simulink model "test_monoaxial"  (R2023a)
settings: Solver=FixedStepAuto  StartTime=0.0  StopTime=inf  FixedStep=0.01  RelTol=1e-3  EnableMultiTasking=on
values from neighbouring files (symbols this model uses):
  A = [Ts 0;Ts Ts]    [monoaxial.m]
  B = [1;0]    [monoaxial.m]
  C = [1,0]    [monoaxial.m]
  D = 0    [monoaxial.m]
undefined symbols (not defined in the file or in its folder): dev, Discrete, Main, pwm_output0, Time
libraries: px4Sensorslib x4, px4lib x1, px4uORBlib x1, ctrlSharedLib x1, slpidlib x1
settings Model: SimulationMode=external  ExtModeTrigDuration=10  Creator=ArriGE66  LastModifiedBy=User
settings SolverCC: PositivePriorityOrder=on
settings OptimizationCC: EnhancedBackFolding=on  PassReuseOutputArgsAs=Individual arguments  ZeroExternalMemoryAtStartup=off  ZeroInternalMemoryAtStartup=off  MaxStackSize=64  OptimizeBlockOrder=speed  DifferentSizesBufferReuse=on  OptimizationCustomize=off  EfficientTunableParamExpr=on
settings DebuggingCC: ParameterTunabilityLossMsg=error
settings HardwareCC: ProdBitPerPointer=32  ProdBitPerSizeT=32  ProdBitPerPtrDiffT=32  ProdLargestAtomicInteger=Long  ProdLargestAtomicFloat=Double  ProdWordSize=32  ProdLongLongMode=on  ProdHWDeviceType=ARM Compatible->ARM Cortex
settings SFSimCC: MATLABDynamicMemAlloc=off  SimTargetLang=C++
settings RTWCC: Description=Embedded Coder  SystemTargetFile=ert.tlc  HardwareBoard=PX4 Cube Orange  TemplateMakefile=ert_default_tmf  Toolchain=GNU Tools for PX4 Autopilots  TargetLang=C++
settings CodeAppCC: ForceParamTrailComments=on  IgnoreCustomStorageClasses=off  OperatorAnnotations=on  SimulinkDataObjDesc=on  SFDataObjDesc=on  InsertBlockDesc=on
settings ERTTargetCC: ExtMode=on  ExtModeTransport=3  ExtModeStaticAlloc=on  ExtModeStaticAllocSize=1024  ExtModeMexFile=ext_xcp  ExtModeMexArgs=1 COM10 3000000  ExtModeIntrfLevel=Level2 - Open

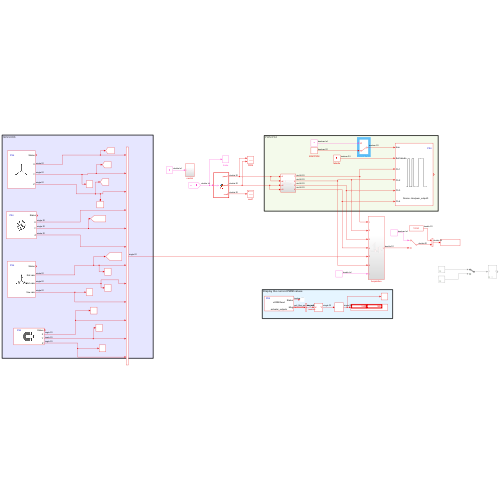
[thumbnail: Simulink's stored preview of the top-level diagram]
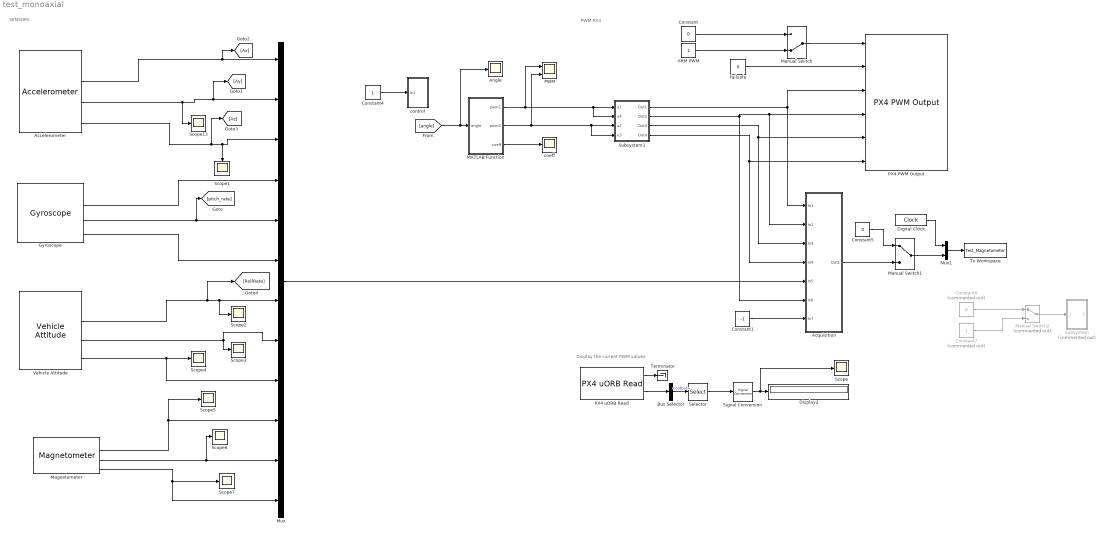
== system test_monoaxial ==
  note: PWM PX4
  note: SENSORS
  note: Display the current PWM values
  ARM PWM : Constant  OutDataTypeStr=boolean  SampleTime=0.01
  Accelerometer : px4Sensorslib/Accelerometer  uorbTimeStamp=off  BlockingMode=off  BlockTimeout=1e-3  sampleTime=1/100
  Acquisition : Subsystem
  Angle : Scope
  Bus Selector : BusSelector  OutputSignals=output
  Constant : Constant  Value=0  OutDataTypeStr=boolean
  Constant1 : Constant  Value=-1
  Constant4 : Constant
  Constant5 : Constant  Value=0  OutDataTypeStr=boolean
  Constant6 : Constant  Commented=on  Value=0
  Constant7 : Constant  Commented=on
  Digital Clock : DigitalClock  SampleTime=-1
  Display2 : Display
  Gyroscope : px4Sensorslib/Gyroscope  uorbTimeStamp=off  BlockingMode=off  BlockTimeout=1e-3  sampleTime=1/100
  MATLAB Function : MATLAB Function  TreatAsAtomicUnit=on
  Magnetometer : px4Sensorslib/Magnetometer  uorbTimeStamp=off  BlockingMode=off  BlockTimeout=1e-3  sampleTime=0.01
  Manual Switch : ManualSwitch  CurrentSetting=0
  Manual Switch1 : ManualSwitch
  Manual Switch2 : ManualSwitch  Commented=on
  Mux : Mux  Inputs=12
  Mux1 : Mux  Inputs=2
  PWM : Scope  NumInputPorts=2
  PX4 PWM Output : px4lib/PX4 PWM Output  pwmDevice=Main (/dev/pwm_output0)  pwmChannel1_=on  pwmChannel2_=on  pwmChannel3_=on  pwmChannel4_=on  pwmChannel5_=off  pwmChannel6_=off  pwmChannel7_=off  pwmChannel8_=off  forceTerminateFailsafe=off  outputErrorStatus=on
  PX4 uORB Read : px4uORBlib/PX4 uORB Read  uORBTopic=actuator_outputs  selectInstance=actuator_outputs  SampleTime=0.01  BlockingMode=off  BlockTimeout=1e-3
  Scope{,1..7,13} (9 alike) : Scope
  Selector : Selector  InputPortWidth=16  IndexOptions=Index vector (dialog)  Indices=[1 2]  OutputSizes=1
  Signal Conversion : SignalConversion  OverrideOpt=off
  Subsystem : Subsystem  Commented=on  mask{delta_t=10}
      mask prompts: delta_t "delta_time [s]"
  Subsystem1 : Subsystem
  Terminator : Terminator
  To Workspace : ToWorkspace  VariableName=Test_Magnetometer  SampleTime=-1
      settings: Save2DSignal=2-D array (concatenate along first dimension)
  Vehicle Attitude : px4Sensorslib/Vehicle Attitude  rollRate=on  pitchRate=on  yawRate=on  quaternion=off  uorbTimeStamp=off  BlockingMode=off  BlockTimeout=0.001  sampleTime=1/100
  coeff : Scope
  control : Subsystem
  failsafe : Constant  Value=0  OutDataTypeStr=boolean  SampleTime=0.01
  wires:
  Manual Switch/1 -> PX4 PWM Output/1
  Bus Selector/1 -> Selector/1  "<output>"
  PX4 uORB Read/1 -> Terminator/1
  failsafe/1 -> PX4 PWM Output/2
  Selector/1 -> Signal Conversion/1
  PX4 uORB Read/2 -> Bus Selector/1
  Signal Conversion/1 -> Scope/1, Display2/1
  Vehicle Attitude/3 -> Scope3/1, Mux/8
  Vehicle Attitude/2 -> [RollRate], Scope2/1, Mux/7
  ARM PWM/1 -> Manual Switch/2
  Constant/1 -> Manual Switch/1
  Gyroscope/4 -> Mux/6
  Gyroscope/3 -> [pitch_rate], Mux/5
  Gyroscope/2 -> Mux/4
  Accelerometer/2 -> [Ax], Mux/1
  Accelerometer/3 -> Scope13/1, [Ay], Mux/2
  Accelerometer/4 -> [Az], Mux/3, Scope1/1
  Mux/1 -> Acquisition/5(In5)
  Acquisition/1(Out1) -> Manual Switch1/2
  Constant5/1 -> Manual Switch1/1
  Mux1/1 -> To Workspace/1
  Digital Clock/1 -> Mux1/1
  Manual Switch1/1 -> Mux1/2
  Constant7/1 -> Manual Switch2/2
  Constant6/1 -> Manual Switch2/1
  Manual Switch2/1 -> Subsystem/1(In1)
  Vehicle Attitude/4 -> Mux/9, Scope4/1
  Subsystem1/2(Out2) -> Acquisition/6(In6), Acquisition/2(In2), PX4 PWM Output/4
  Subsystem1/3(Out3) -> Acquisition/3(In3), PX4 PWM Output/5
  Subsystem1/1(Out1) -> Acquisition/1(In1), PX4 PWM Output/3
  Subsystem1/4(Out4) -> Acquisition/4(In4), PX4 PWM Output/6
  Magnetometer/2 -> Mux/10, Scope5/1
  Magnetometer/3 -> Mux/11, Scope6/1
  Magnetometer/4 -> Mux/12, Scope7/1
  Constant1/1 -> Acquisition/7(In7)
  [angle] -> MATLAB Function/1(angle), Angle/1
  MATLAB Function/1(pwm1) -> Subsystem1/2(u4), Subsystem1/1(u1), PWM/1
  MATLAB Function/3(coeff) -> coeff/1
  Constant4/1 -> control/1(In1)
  MATLAB Function/2(pwm2) -> Subsystem1/4(u3), Subsystem1/3(u2), PWM/2

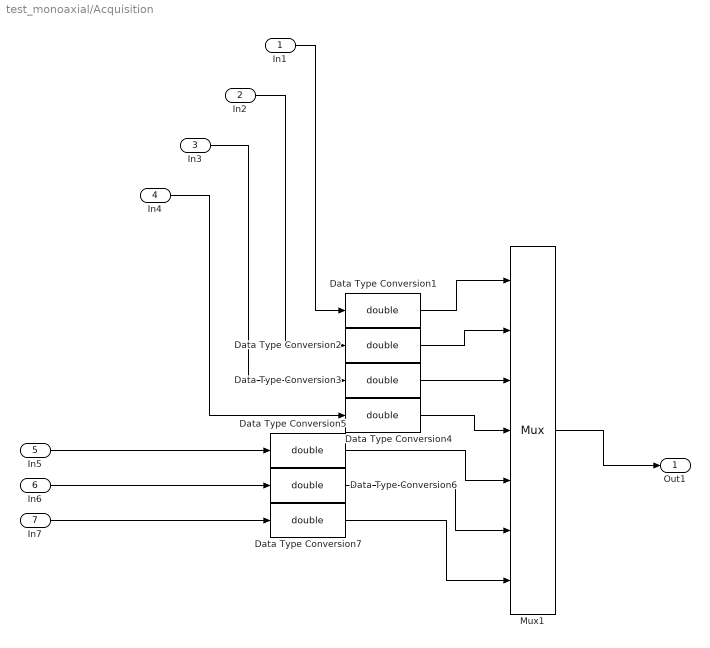
== system test_monoaxial/Acquisition ==
  In1 : Inport
  In2 : Inport  Port=2
  In3 : Inport  Port=3
  In4 : Inport  Port=4
  In5 : Inport  Port=5
  In6 : Inport  Port=6
  In7 : Inport  Port=7
  Data Type Conversion{1..7} (7 alike) : DataTypeConversion  OutDataTypeStr=double  SaturateOnIntegerOverflow=off  RndMeth=Floor
  Mux1 : Mux  Inputs=7
      settings: DisplayOption=signals
  Out1 : Outport
  wires:
  In7/1 -> Data Type Conversion7/1
  In2/1 -> Data Type Conversion2/1
  Data Type Conversion1/1 -> Mux1/1
  Data Type Conversion7/1 -> Mux1/7
  Data Type Conversion3/1 -> Mux1/3
  Data Type Conversion5/1 -> Mux1/5
  Data Type Conversion4/1 -> Mux1/4
  Data Type Conversion2/1 -> Mux1/2
  Data Type Conversion6/1 -> Mux1/6
  In3/1 -> Data Type Conversion3/1
  In6/1 -> Data Type Conversion6/1
  Mux1/1 -> Out1/1
  In5/1 -> Data Type Conversion5/1
  In1/1 -> Data Type Conversion1/1
  In4/1 -> Data Type Conversion4/1

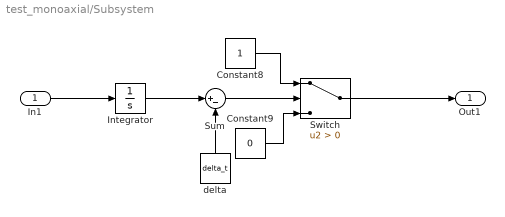
== system test_monoaxial/Subsystem ==
  In1 : Inport
  Constant8 : Constant
  Constant9 : Constant  Value=0
  Integrator : Integrator
  Sum : Sum  Inputs=|+-
  Switch : Switch  Criteria=u2 > Threshold  SaturateOnIntegerOverflow=off  InputSameDT=off
  delta : Constant  Value=delta_t
  Out1 : Outport
  wires:
  delta/1 -> Sum/2
  In1/1 -> Integrator/1
  Sum/1 -> Switch/2
  Integrator/1 -> Sum/1
  Switch/1 -> Out1/1
  Constant9/1 -> Switch/3
  Constant8/1 -> Switch/1

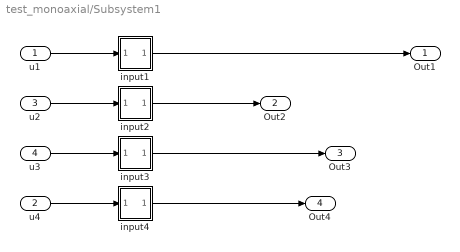
== system test_monoaxial/Subsystem1 ==
  u1 : Inport
  u4 : Inport  Port=2
  u2 : Inport  Port=3
  u3 : Inport  Port=4
  input1 : Subsystem
  input2 : Subsystem
  input3 : Subsystem
  input4 : Subsystem
  Out1 : Outport
  Out2 : Outport  Port=2
  Out3 : Outport  Port=3
  Out4 : Outport  Port=4
  wires:
  u2/1 -> input2/1(In1)
  u1/1 -> input1/1(In1)
  input1/1(Out1) -> Out1/1
  u4/1 -> input4/1(In1)
  input4/1(Out1) -> Out4/1
  input2/1(Out1) -> Out2/1
  u3/1 -> input3/1(In1)
  input3/1(Out1) -> Out3/1

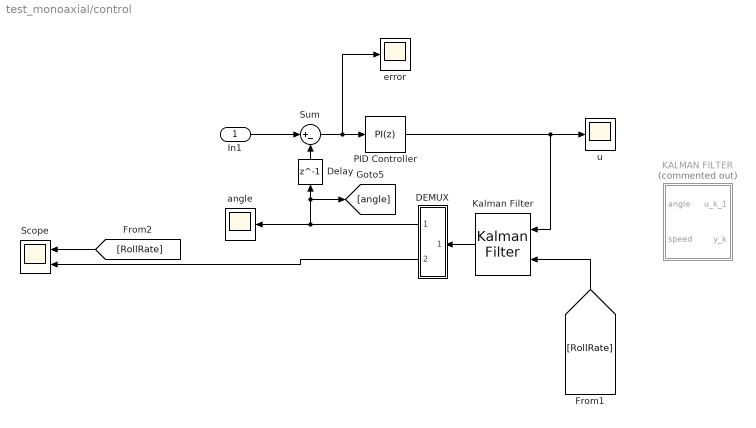
== system test_monoaxial/control ==
  In1 : Inport
  DEMUX : MATLAB Function  TreatAsAtomicUnit=on
  Delay : Delay  DelayLength=1
  KALMAN FILTER : Subsystem  Commented=on
  Kalman Filter : ctrlSharedLib/Kalman Filter  TimeDomain=Discrete-Time  UseCurrentEstimator=on  ModelSource=Individual A, B, C, D matrices  ModelSourceVariable=ss(0.95,1,1,0,1)  A=A  B=B  C=C  D=D  NumberOfStates=1  NumberOfInputs=1  NumberOfOutputs=1  InitialEstimateSource=Dialog  X0=0  P0=10  UseK=off  UseGH=off  NumberOfProcessNoiseInputs=1  G=1  TimeInvariantG=on  H=0  TimeInvariantH=on  Q=10  TimeInvariantQ=on  R=0.01  TimeInvariantR=on  N=0  TimeInvariantN=on  AddInputPort=on  AddEnablePort=off  OutputEstimatedY=off  OutputP=off  Ts=-1
  PID Controller : slpidlib/PID Controller  Controller=PI  Form=Parallel  TimeDomain=Discrete-time  UseExternalTs=off  SampleTime=-1  IntegratorMethod=Forward Euler  FilterMethod=Forward Euler  ControllerParametersSource=internal  P=14.044  I=209.05  UseKiTs=off  D=0  N=100  UseFilter=on  TunerSelectOption=Transfer Function Based (PID Tuner App)  InitialConditionSource=internal  InitialConditionForIntegrator=0  InitialConditionForFilter=0  DifferentiatorICPrevScaledInput=0  ExternalReset=none  TrackingMode=off  Kt=1  LimitOutput=off  SatLimitsSource=internal  UpperSaturationLimit=inf  LowerSaturationLimit=-inf  LinearizeAsGain=on  AntiWindupMode=none  Kb=1  LimitIntegrator=off  UpperIntegratorSaturationLimit=inf  LowerIntegratorSaturationLimit=-inf  POutMin=[]  POutMax=[]  IOutMin=[]  IOutMax=[]  DOutMin=[]  DOutMax=[]  NOutMin=[]  NOutMax=[]  SumOutMin=[]  SumOutMax=[]  SaturationOutMin=[]  SaturationOutMax=[]  PParamMin=[]  PParamMax=[]  IParamMin=[]  IParamMax=[]  DParamMin=[]  DParamMax=[]  NParamMin=[]  NParamMax=[]  KbParamMin=[]  KbParamMax=[]  KtParamMin=[]  KtParamMax=[]  KbOutMin=[]  KbOutMax=[]  KtOutMin=[]  KtOutMax=[]  IntegratorOutMin=[]  IntegratorOutMax=[]  FilterOutMin=[]  FilterOutMax=[]  SumI1OutMin=[]  SumI1OutMax=[]  SumI2OutMin=[]  SumI2OutMax=[]  SumI3OutMin=[]  SumI3OutMax=[]  SumI4OutMin=[]  SumI4OutMax=[]  SumDOutMin=[]  SumDOutMax=[]  DifferentiatorOutMin=[]  DifferentiatorOutMax=[]  FilterDiffOutCoefMin=[]  FilterDiffOutCoefMax=[]  ReciprocalOutMin=[]  ReciprocalOutMax=[]  SumDenOutMin=[]  SumDenOutMax=[]  SumNumOutMin=[]  SumNumOutMax=[]  DivideOutMin=[]  DivideOutMax=[]  UdiffTsProdOutMin=[]  UdiffTsProdOutMax=[]  NTsProdOutMin=[]  NTsProdOutMax=[]  UintegralTsProdOutMin=[]  UintegralTsProdOutMax=[]  UngainTsProdOutMin=[]  UngainTsProdOutMax=[]  ClampingZeroOutDataTypeStr=Inherit: Inherit via back propagation  ClampingZeroOutMin=[]  ClampingZeroOutMax=[]  FilterDenConstantOutDataTypeStr=Inherit: Inherit via back propagation  FilterDenConstantOutMin=[]  FilterDenConstantOutMax=[]  PCopyOutDataTypeStr=Inherit: Inherit via back propagation  PCopyOutMin=[]  PCopyOutMax=[]  NCopyOutDataTypeStr=Inherit: Inherit via back propagation  NCopyOutMin=[]  NCopyOutMax=[]  IntegratorContinuousStateAttributes=''  IntegratorStateMustResolveToSignalObject=off  IntegratorRTWStateStorageClass=Auto  FilterContinuousStateAttributes=''  FilterStateMustResolveToSignalObject=off  FilterRTWStateStorageClass=Auto  ParallelPVariant=InternalParameters  IdealPVariant=Disabled  IVariant=InternalParameters  DVariant=Disabled  IntegratorVariant=Discrete  SatVariant=Disabled  AWVariant=Passthrough  PCopyVariant=Disabled  TRVariant=Disabled  FdbkBlocksVariant=Forward  IdealPFdbkVariant=Disabled  SatFdbkVariant=Disabled  DerivativeFilterVariant=Disabled  NVariant=Disabled  NCopyVariant=Disabled_SignalSpec  FilterICVariant=Disabled  IntegratorICVariant=InternalICs  ExternalResetVariant=Disabled  TRSumVariant=Passthrough  SumFdbkVariant=Disabled  SumVariant=Sum_PI  TsampFilterVariant=InternalTs  TsampNgainVariant=Passthrough  TsampIntegralVariant=Disabled_SignalSpec  ExternalSaturationOutDataTypeStr=Inherit: Same as second input
  Scope : Scope  NumInputPorts=2
  Sum : Sum  Inputs=|+-
  angle : Scope
  error : Scope
  u : Scope
  wires:
  Sum/1 -> error/1, PID Controller/1
  DEMUX/1(angle) -> angle/1, Delay/1, [angle]
  In1/1 -> Sum/1
  PID Controller/1 -> Kalman Filter/1, u/1
  [RollRate] -> Scope/1
  DEMUX/2(speed) -> Scope/2
  [RollRate] -> Kalman Filter/2
  Delay/1 -> Sum/2
  Kalman Filter/1 -> DEMUX/1(x)

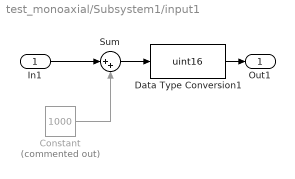
== system test_monoaxial/Subsystem1/input1 ==
  In1 : Inport
  Constant : Constant  Commented=on  Value=1000  SampleTime=0.01
  Data Type Conversion1 : DataTypeConversion  OutDataTypeStr=uint16  SaturateOnIntegerOverflow=off  RndMeth=Floor
  Sum : Sum  Inputs=|++
  Out1 : Outport
  wires:
  Sum/1 -> Data Type Conversion1/1
  In1/1 -> Sum/1
  Constant/1 -> Sum/2
  Data Type Conversion1/1 -> Out1/1

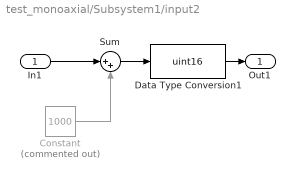
== system test_monoaxial/Subsystem1/input2 ==
  In1 : Inport
  Constant : Constant  Commented=on  Value=1000  SampleTime=0.01
  Data Type Conversion1 : DataTypeConversion  OutDataTypeStr=uint16  SaturateOnIntegerOverflow=off  RndMeth=Floor
  Sum : Sum  Inputs=|++
  Out1 : Outport
  wires:
  Sum/1 -> Data Type Conversion1/1
  In1/1 -> Sum/1
  Constant/1 -> Sum/2
  Data Type Conversion1/1 -> Out1/1

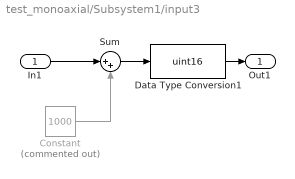
== system test_monoaxial/Subsystem1/input3 ==
  In1 : Inport
  Constant : Constant  Commented=on  Value=1000  SampleTime=0.01
  Data Type Conversion1 : DataTypeConversion  OutDataTypeStr=uint16  SaturateOnIntegerOverflow=off  RndMeth=Floor
  Sum : Sum  Inputs=|++
  Out1 : Outport
  wires:
  Sum/1 -> Data Type Conversion1/1
  In1/1 -> Sum/1
  Constant/1 -> Sum/2
  Data Type Conversion1/1 -> Out1/1

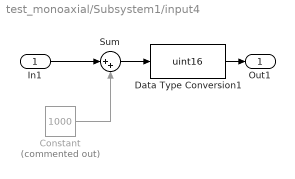
== system test_monoaxial/Subsystem1/input4 ==
  In1 : Inport
  Constant : Constant  Commented=on  Value=1000  SampleTime=0.01
  Data Type Conversion1 : DataTypeConversion  OutDataTypeStr=uint16  SaturateOnIntegerOverflow=off  RndMeth=Floor
  Sum : Sum  Inputs=|++
  Out1 : Outport
  wires:
  Sum/1 -> Data Type Conversion1/1
  In1/1 -> Sum/1
  Constant/1 -> Sum/2
  Data Type Conversion1/1 -> Out1/1

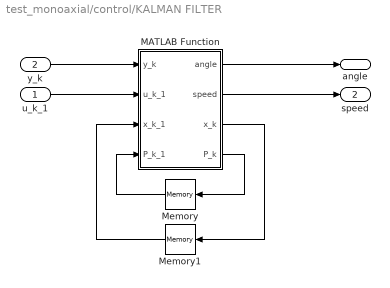
== system test_monoaxial/control/KALMAN FILTER ==
  u_k_1 : Inport
  y_k : Inport  Port=2
  MATLAB Function : MATLAB Function  TreatAsAtomicUnit=on
  Memory : Memory  InheritSampleTime=on  LinearizeAsDelay=on
  Memory1 : Memory  InheritSampleTime=on  LinearizeAsDelay=on
  angle : Outport
  speed : Outport  Port=2
  wires:
  Memory1/1 -> MATLAB Function/3(x_k_1)
  y_k/1 -> MATLAB Function/1(y_k)
  u_k_1/1 -> MATLAB Function/2(u_k_1)
  Memory/1 -> MATLAB Function/4(P_k_1)
  MATLAB Function/1(angle) -> angle/1
  MATLAB Function/2(speed) -> speed/1
  MATLAB Function/3(x_k) -> Memory1/1
  MATLAB Function/4(P_k) -> Memory/1

== matlab function test_monoaxial/control/KALMAN FILTER/MATLAB Function ==
  data: angle output; speed output; y_k input; x_k output; u_k_1 input; x_k_1 input; P_k_1 input; P_k output
function [angle, speed,x_k, P_k] = fcn(y_k, u_k_1,x_k_1, P_k_1)

%PARAMETERS
Ts = 0.01;
R = 0.01;
Q = 10;

A = [Ts 0;Ts Ts];
B = [1;0];
C = [1,0];
D = 0;

P_k = A*P_k_1*A'+Q;
L_k = P_k*C'*(C*P_k*C'+R)^(-1);

x_k = A*x_k_1+B*u_k_1+L_k*(y_k-C*(A*x_k_1+B*u_k_1));
angle = x_k(2,2);
speed = x_k(1,1);

== matlab function test_monoaxial/MATLAB Function ==
  data: angle input; pwm1 output; pwm2 output; coeff output
function [pwm1,pwm2,coeff] = fcn(angle)

max_angle = pi/4;
coeff = 0.5 + (angle/max_angle)/2;

pwm1 = 1000*(1-coeff)+1000;
pwm2 = 1000*coeff + 1000;

== matlab function test_monoaxial/control/DEMUX ==
  data: x input; angle output; speed output
function [angle,speed] = fcn(x)

angle = x(2);
speed = x(1);
